simulink model "battery_boost_regulator_Heating_Load"  (Simulink 9.3)
settings: Solver=ode23t  StartTime=0.0  StopTime=1  MaxStep=1e-6  MinStep=0.5e-6  RelTol=1e-6  AbsTol=1e-6  EnableMultiTasking=on
libraries: powerlib x14, powerlib_extras x1, simulink x1
settings Model: Creator=ruxi  LastModifiedBy=Dominion
settings SolverCC: AutoScaleAbsTol=off  AlgebraicLoopSolver=LineSearch
settings DataIOCC: LimitDataPoints=on
settings OptimizationCC: ExpressionDepthLimit=2147483647  InitFltsAndDblsToZero=on
settings DebuggingCC: SaveWithParameterizedLinksMsg=none  SignalResolutionControl=TryResolveAllWithWarning  SolverPrmCheckMsg=warning  MultiTaskDSMMsg=warning  MultiTaskCondExecSysMsg=none  StateNameClashWarn=warning
settings SFSimCC: SimUseLocalCustomCode=on
settings RTWCC: RTWUseLocalCustomCode=on
settings GRTTargetCC: TargetFcnLib=ansi_tfl_tmw.mat
settings ConfigComp: CovExternalEMLEnable=on

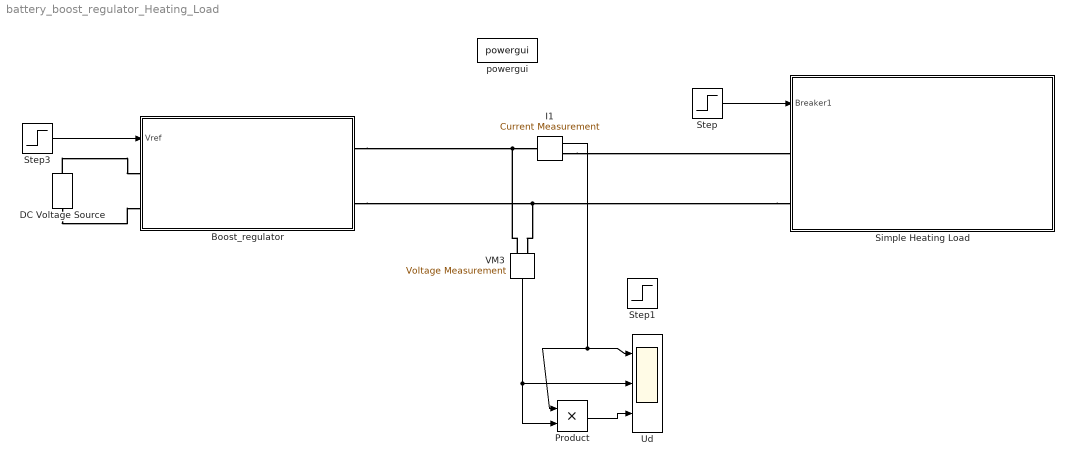
== system battery_boost_regulator_Heating_Load ==
  Boost_regulator : Subsystem
  DC Voltage Source : powerlib/Electrical Sources/DC Voltage Source  Amplitude=45  Measurements=None
      settings: SourceProductName=Simscape Electrical
  I1 : powerlib/Measurements/Current Measurement  Tag=PoWeRsYsTeMmEaSuReMeNt  PhasorSimulation=off  OutputType=Magnitude  PSBequivalent=0
      settings: SourceProductName=Simscape Electrical
  Product : Product  RndMeth=Zero
  Simple Heating Load : Subsystem
  Step : Step  Time=0.1  SampleTime=0
  Step1 : Step  Time=0.3  SampleTime=0
  Step3 : Step  Time=0  After=300  SampleTime=0
  Ud : Scope  NumInputPorts=3
  VM3 : powerlib/Measurements/Voltage Measurement  PhasorSimulation=off  OutputType=Complex  PSBequivalent=0
      settings: SourceProductName=Simscape Electrical
  powergui : powerlib/powergui  SimulationMode=Discrete  SampleTime=1e-5  frequency=60  Iterations=50  frequencyindice=0  Pbase=100e6  ErrMax=1e-4  UnitsV=kV  UnitsW=MW  buscounter=0  FunctionMessages=off  echomessages=off  EnableUseOfTLC=off  CurrentSourceSwitches=off  DisableSnubberDevices=off  DisableRonSwitches=off  DisableVfSwitches=off  DisplayEquations=off  AutomaticDiscreteSolvers=off  SolverType=Tustin/Backward Euler (TBE)  Interpol=off  ExternalGateDelay=off  methode=off  Ts=0  x0status=blocks  SPID=on  SwTol=0  HookPort=off  NonlinearTolerance=0  nMaxIteration=15  ContinueOnMaxIteration=off  RestoreLinks=warning  ResistiveCurrentMeasurement=off  Frange=[0:2:500]  Ylog=off  Xlog=on  ShowGrid=off  save=off  variable=ZData  structure=0  ZoomFFT=on  StartTime=0.0  cycles=1  DisplayStyle=1  fundamental=60  FreqAxis=off  MaxFrequency=1000  frequencyindicesteady=1  RmsSteady=1  display=off
      settings: SourceProductName=Simscape Electrical
  wires:
  Step/1 -> Simple Heating Load/1(Breaker1)
  I1/1 -> Ud/1, Product/1
  VM3/1 -> Ud/2, Product/2
  Product/1 -> Ud/3
  Step3/1 -> Boost_regulator/1(Vref)
  connections:
  VM3/LConn1 -- Boost_regulator/RConn1 -- I1/LConn1
  Simple Heating Load/LConn2 -- Boost_regulator/RConn2 -- VM3/LConn2
  I1/RConn1 -- Simple Heating Load/LConn1
  DC Voltage Source/RConn1 -- Boost_regulator/LConn1
  DC Voltage Source/LConn1 -- Boost_regulator/LConn2

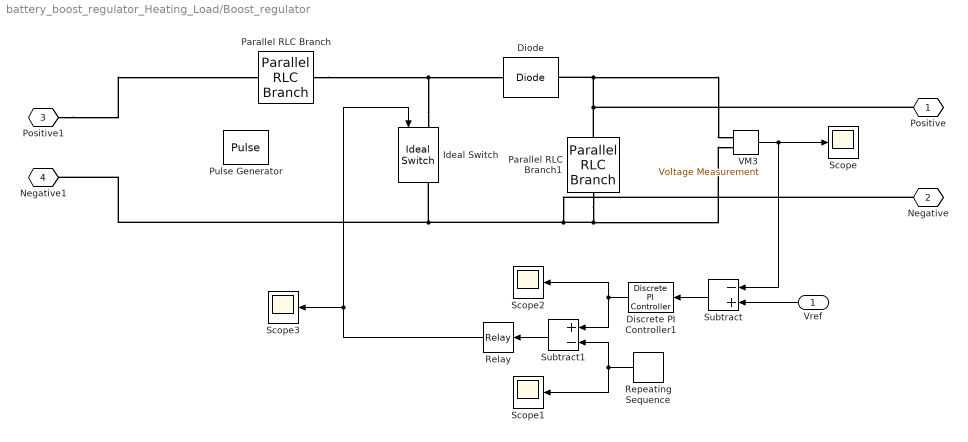
== system battery_boost_regulator_Heating_Load/Boost_regulator ==
  Vref : Inport
  Diode : powerlib/Power Electronics/Diode  Ron=0.001  Lon=0  Vf=0  IC=0  UseSnubber=0  Rs=50000  Cs=250e-9  Measurements=off
      settings: SourceProductName=Simscape Electrical
  Discrete PI Controller1 : powerlib_extras/Discrete  Control Blocks/Discrete PI Controller  Kp=0.001  Ki=0.2  Par_Limits=[10 -10]  Init=0  Ts=1e-6
      settings: SourceProductName=Simscape Electrical
  Ideal Switch : powerlib/Power Electronics/Ideal Switch  Ron=0.001  Lon=0  IC=0  Rs=1e5  Cs=inf  Measurements=on
      settings: SourceProductName=Simscape Electrical
  Parallel RLC Branch : powerlib/Elements/Parallel RLC Branch  LConnTagsString=a  RConnTagsString=__new0  BranchType=L  Resistance=1  Inductance=1e-3  SetiL0=off  InitialCurrent=0  Capacitance=1e-6  Setx0=off  InitialVoltage=0  Measurements=None
      settings: SourceProductName=Simscape Electrical
  Parallel RLC Branch1 : powerlib/Elements/Parallel RLC Branch  LConnTagsString=a  RConnTagsString=__new0  BranchType=C  Resistance=1  Inductance=1e-3  SetiL0=off  InitialCurrent=0  Capacitance=1e-3  Setx0=on  InitialVoltage=100  Measurements=None
      settings: SourceProductName=Simscape Electrical
  Pulse Generator : DiscretePulseGenerator  PulseType=Time based  Period=1e-3  PulseWidth=90
  Relay : Relay  OnSwitchValue=0.01  OffSwitchValue=-0.01
  Repeating Sequence : simulink/Sources/Repeating Sequence  rep_seq_t=[0 1e-3 2e-3]  rep_seq_y=[-10 10 -10]
  Scope{,1..3} (4 alike) : Scope
  Subtract : Sum  Inputs=-+
  Subtract1 : Sum  Inputs=+-
  VM3 : powerlib/Measurements/Voltage Measurement  PhasorSimulation=off  OutputType=Complex  PSBequivalent=0
      settings: SourceProductName=Simscape Electrical
  Positive : PMIOPort  Tag=PMCPort  Side=Right
  Negative : PMIOPort  Tag=PMCPort  Port=2  Side=Right
  Positive1 : PMIOPort  Tag=PMCPort  Port=3  Side=Left
  Negative1 : PMIOPort  Tag=PMCPort  Port=4  Side=Left
  wires:
  VM3/1 -> Scope/1, Subtract/1
  Vref/1 -> Subtract/2
  Subtract/1 -> Discrete PI Controller1/1
  Discrete PI Controller1/1 -> Subtract1/1, Scope2/1
  Repeating Sequence/1 -> Subtract1/2, Scope1/1
  Subtract1/1 -> Relay/1
  Relay/1 -> Ideal Switch/1, Scope3/1
  connections:
  Ideal Switch/LConn1 -- Parallel RLC Branch/LConn1 -- Diode/LConn1
  Parallel RLC Branch1/LConn1 -- Diode/RConn1 -- VM3/LConn1 -- Positive/RConn1
  Negative1/RConn1 -- Ideal Switch/RConn1 -- VM3/LConn2 -- Parallel RLC Branch1/RConn1 -- Negative/RConn1
  Positive1/RConn1 -- Parallel RLC Branch/RConn1

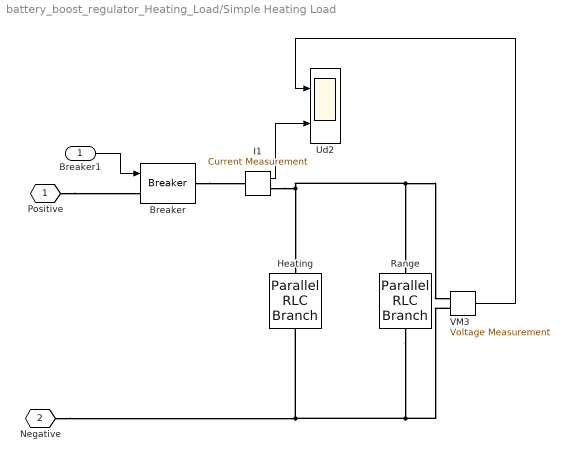
== system battery_boost_regulator_Heating_Load/Simple Heating Load ==
  Breaker1 : Inport
  Breaker : powerlib/Elements/Breaker  InitialState=0  SwitchingTimes="[ 1/60  5/60 ]"  External=on  BreakerResistance=0.01  SnubberResistance=1e6  SnubberCapacitance=inf  Measurements=None  MoreParameters=off  NoBreakLoop=off
      settings: SourceProductName=Simscape Electrical
  Heating : powerlib/Elements/Parallel RLC Branch  LConnTagsString=a  RConnTagsString=__new0  BranchType=R  Resistance=90  Inductance=1e-3  SetiL0=off  InitialCurrent=0  Capacitance=1e-6  Setx0=off  InitialVoltage=0  Measurements=None
      settings: SourceProductName=Simscape Electrical
  I1 : powerlib/Measurements/Current Measurement  Tag=PoWeRsYsTeMmEaSuReMeNt  PhasorSimulation=off  OutputType=Magnitude  PSBequivalent=0
      settings: SourceProductName=Simscape Electrical
  Range : powerlib/Elements/Parallel RLC Branch  LConnTagsString=a  RConnTagsString=__new0  BranchType=R  Resistance=90  Inductance=1e-3  SetiL0=off  InitialCurrent=0  Capacitance=1e-6  Setx0=off  InitialVoltage=0  Measurements=None
      settings: SourceProductName=Simscape Electrical
  Ud2 : Scope  NumInputPorts=2
  VM3 : powerlib/Measurements/Voltage Measurement  PhasorSimulation=off  OutputType=Complex  PSBequivalent=0
      settings: SourceProductName=Simscape Electrical
  Positive : PMIOPort  Tag=PMCPort  Side=Left
  Negative : PMIOPort  Tag=PMCPort  Port=2  Side=Left
  wires:
  I1/1 -> Ud2/2
  VM3/1 -> Ud2/1
  Breaker1/1 -> Breaker/1
  connections:
  VM3/LConn1 -- Heating/LConn1 -- I1/RConn1 -- Range/LConn1
  VM3/LConn2 -- Negative/RConn1 -- Heating/RConn1 -- Range/RConn1
  Breaker/RConn1 -- I1/LConn1
  Positive/RConn1 -- Breaker/LConn1
